simulink model "transmitancje_dyskretne"  (R2018b)
settings: Solver=VariableStepAuto  StartTime=0.0  StopTime=10.0  RelTol=1e-3
settings Model: Creator=mariu  LastModifiedBy=mariu

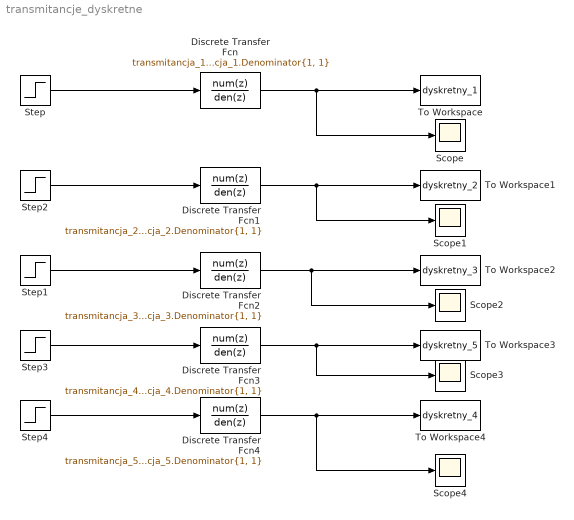
== system transmitancje_dyskretne ==
  Discrete Transfer Fcn : DiscreteTransferFcn  Numerator=transmitancja_1.Numerator{1, 1}  Denominator=transmitancja_1.Denominator{1, 1}
  Discrete Transfer Fcn1 : DiscreteTransferFcn  Numerator=transmitancja_2.Numerator{1, 1}  Denominator=transmitancja_2.Denominator{1, 1}
  Discrete Transfer Fcn2 : DiscreteTransferFcn  Numerator=transmitancja_3.Numerator{1, 1}  Denominator=transmitancja_3.Denominator{1, 1}
  Discrete Transfer Fcn3 : DiscreteTransferFcn  Numerator=transmitancja_4.Numerator{1, 1}  Denominator=transmitancja_4.Denominator{1, 1}
  Discrete Transfer Fcn4 : DiscreteTransferFcn  Numerator=transmitancja_5.Numerator{1, 1}  Denominator=transmitancja_5.Denominator{1, 1}
  Scope{,1..4} (5 alike) : Scope
  Step{,1..4} (5 alike) : Step  SampleTime=0
  To Workspace : ToWorkspace  VariableName=dyskretny_1  SaveFormat=Timeseries  SampleTime=-1
  To Workspace1 : ToWorkspace  VariableName=dyskretny_2  SaveFormat=Timeseries  SampleTime=-1
  To Workspace2 : ToWorkspace  VariableName=dyskretny_3  SaveFormat=Timeseries  SampleTime=-1
  To Workspace3 : ToWorkspace  VariableName=dyskretny_5  SaveFormat=Timeseries  SampleTime=-1
  To Workspace4 : ToWorkspace  VariableName=dyskretny_4  SaveFormat=Timeseries  SampleTime=-1
  wires:
  Discrete Transfer Fcn/1 -> Scope/1, To Workspace/1
  Step/1 -> Discrete Transfer Fcn/1
  Step4/1 -> Discrete Transfer Fcn4/1
  Step3/1 -> Discrete Transfer Fcn3/1
  Step1/1 -> Discrete Transfer Fcn2/1
  Step2/1 -> Discrete Transfer Fcn1/1
  Discrete Transfer Fcn1/1 -> Scope1/1, To Workspace1/1
  Discrete Transfer Fcn2/1 -> Scope2/1, To Workspace2/1
  Discrete Transfer Fcn3/1 -> Scope3/1, To Workspace3/1
  Discrete Transfer Fcn4/1 -> Scope4/1, To Workspace4/1
